simulink model "VFlexP"  (R2024a)
settings: Solver=ode23tb  StartTime=0.0  StopTime=3  FixedStep=1e-5
model workspace (MAT data in the model file):
  DCop_DCBUCK : object (value not decoded)
  Grid_CCVSC_idx = [2; 3; 4; 5; 6; 7; 8; 9; 10; 11; 12]
  Grid_CCVSCs = 1
  Grid_CCVSCs_buses = 1
  Grid_CCVSCs_toM = [0 1 0 0 0 0 0 0 0 0 0 0 ... (781 elements, 71x11)]
  Grid_C_Lines = [0 0]
  Grid_Cbuses = [0.00666666666667 0.00666666666667 0.00666666666667]
  Grid_DC : object (value not decoded)
  Grid_DCop_DCBUCK : object (value not decoded)
  Grid_DCop_DC_PES : object (value not decoded)
  Grid_DFIGs = 1
  Grid_DFIGs_buses = 1
  Grid_DGs : string (value not decoded)
  Grid_From_buses = [1 2]
  Grid_GFls = 1
  Grid_GFls_buses = 1
  Grid_GFr_idx = 1
  Grid_GFrs = 1
  Grid_GFrs_buses = 1
  Grid_GFrs_toM = [1; 0; 0]
  Grid_IG_idx = 2
  Grid_IGs = 1
  Grid_IGs_buses = 1
  Grid_IGs_toM = [0; 1]
  Grid_L_Lines = [0.05 0.05]
  Grid_L_Loads = 0
  Grid_Lines_fromM : object (value not decoded)
  Grid_Lines_toM : object (value not decoded)
  Grid_Load_buses = []
  Grid_Load_busesDC = []
  Grid_MSGs = 1
  Grid_MSGs_buses = 1
  Grid_Nbuses = 3
  Grid_PQ_gen = 3
  Grid_Ploads = []
  Grid_PloadsDC = []
  Grid_Ps_lf = -0.138475313333
  Grid_Qloads = []
  Grid_Qs_lf = 0.00594619333333
  Grid_R_Lines = [0.005 0.005]
  Grid_R_Loads = 0
  Grid_R_Loads_DC = 0
  Grid_Rcf = [150 150 150]
  Grid_SCs = 1
  Grid_SCs_buses = 1
  Grid_SG_idx = 1
  Grid_SGs = 1
  Grid_SGs_buses = 1
  Grid_SGs_toM = [1; 0]
  Grid_To_buses = [2 3]
  Grid_VCVSC_idx = [1; 2; 3; 4; 5; 6; 7; 8; 9; 10; 11; 12]
  Grid_VCVSCs = 1
  Grid_VCVSCs_buses = [1; 2; 3; 6; 8; 9; 12; 58; 59; 60; 63; 65]
  Grid_VCVSCs_toM = [1 0 0 0 0 0 0 0 0 0 0 0 ... (852 elements, 71x12)]
  Grid_VSM_idx = 2
  Grid_VSMs = 1
  Grid_VSMs_buses = 1
  Grid_VSMs_toM = [0; 1]
  Grid_admitt_matrix = [1.9801990198-19.801979198i  -1.9801980198+19.801980198i; -1.9801980198+19.801980198i  1.9801990198-19.801979198i]
  Grid_admitt_matrix_noloads = [1.9801990198-19.801979198i  -1.9801980198+19.801980198i; -1.9801980198+19.801980198i  1.9801990198-19.801979198i]
  Grid_bus = [1; 2; 3]
  Grid_busDC_complexity = 1
  Grid_busDC_complexity_PF = 2
  Grid_bus_complexity = [1 1 1]
  Grid_bus_complexity_PF = [1 1 1]
  Grid_buses_lf = 1
  Grid_conductance_matrix = 0.00666666666667
  Grid_conductance_matrix_noloads = 0.00666666666667
  Grid_fref : object (value not decoded)
  Grid_gen_static_params : mBase (value not decoded)
  Grid_iPs_lf = -7.22150378958
  Grid_iQs_lf = 168.17482109
  Grid_iadmitt_matrix = [250000.001075-249999.987531i  249999.998575-250000.012531i; 249999.998575-250000.012531i  250000.001075-249999.987531i]
  Grid_iadmitt_matrix_noloads = [250000.001075-249999.987531i  249999.998575-250000.012531i; 249999.998575-250000.012531i  250000.001075-249999.987531i]
  Grid_iconductance_matrix = 150
  Grid_iconductance_matrix_noloads = 150
  Grid_init_OK_bool = 1
  Grid_intconv_PF : object (value not decoded)
  Grid_lf_op : op_report (value not decoded)
  Grid_lineDC_complexity = []
  Grid_lineDC_complexity_PF = []
  Grid_line_complexity = [1 1]
  Grid_line_complexity_PF = [3 3]
  Grid_loadDC_complexity = []
  Grid_loadDC_complexity_PF = []
  Grid_load_complexity = []
  Grid_load_complexity_PF = []
  Grid_opDC_CCVSC : object (value not decoded)
  Grid_opDC_VSM : object (value not decoded)
  Grid_opGFr : object (value not decoded)
  Grid_opVCVSC : object (value not decoded)
  Grid_op_CCVSC : object (value not decoded)
  Grid_op_IG : object (value not decoded)
  Grid_op_SG : object (value not decoded)
  Grid_op_VSM : object (value not decoded)
  Grid_shift_lines = [0 0]
  Grid_tap_lines = [1 1]
  Grid_v_buses_mod = [1 1.0001218564 1]
  LinsysParamChangeStruct : Param1 (value not decoded)
  Lline = 0.01
  Rline = 1e-05
  linsys : object (value not decoded)
symbols that are objects in the model workspace (value not decoded): Grid_DCop_DC_PES, Grid_DCop_DCBUCK, Grid_op_CCVSC, Grid_op_IG, Grid_op_SG, Grid_op_VSM, Grid_opDC_CCVSC, Grid_opDC_VSM, Grid_opGFr, Grid_opVCVSC
undefined symbols (not defined in the file or in its folder): block_buses_DC, block_idx, CCVSC_idx, Cf, costs, costs2, DFIGs_nodes, DiscIntNeverNeededParam, entity, Fb, Fi, From_nodes, Grid_op_DFIG, Grid_op_DFIG_PQ, Grid_op_MSG, Grid_op_SC, Grid_op_VCVSC, Kic, Kiv, Kpc, Kpv, last_send, Lc, Lf, m, Matrix_flux_to_i, mD, mp, MSGs_buses, Nbuses_DC, nq, op_VCVSC, Psche, Rc, Rf, rkq1, rkq2, SCs_buses, SCs_nodes, sec_control_structure, set_DG_up, set_extra_satur, set_sending_cost, SGs_buses, SGs_nodes, Tf, To_nodes, VI_L, VI_R, WOF_Tf, xkq1, xkq2
libraries: simulink x447, eeGeneralControl x5
(part 5 of 30)

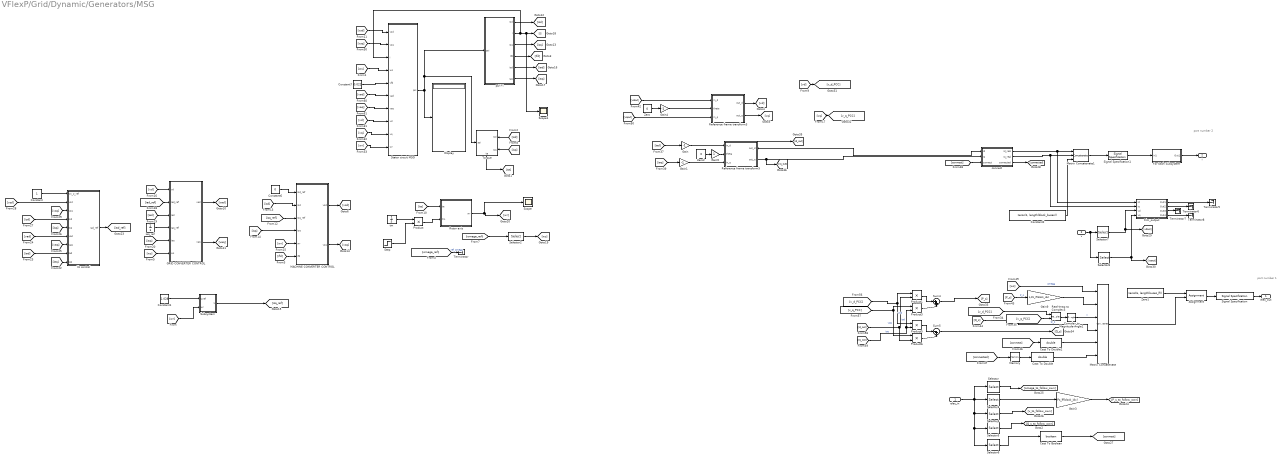
== system VFlexP/Grid/Dynamic/Generators/MSG ==
  note: port number 1
  note: port number 2
  elec_in : Inport
  v : Inport  Port=2
  Assignment : Assignment  NumberOfDimensions=2  DiagnosticForDimensions=Warning  IndexOptions=Assign all,Index vector (dialog)  Indices=1,block_idx  OutputSizes=1,1
  Cast To Boolean : DataTypeConversion  OutDataTypeStr=boolean  SaturateOnIntegerOverflow=off  RndMeth=Floor
  Cast To Double : DataTypeConversion  OutDataTypeStr=double  SaturateOnIntegerOverflow=off  RndMeth=Floor
  Cast To Double1 : DataTypeConversion  OutDataTypeStr=double  SaturateOnIntegerOverflow=off  RndMeth=Floor
  Complex to Magnitude-Angle1 : ComplexToMagnitudeAngle  Output=Magnitude
  Constant : Constant
  Constant1 : Constant  Value=1.028
  Constant2 : Constant  Value=zeros(1, length(block_buses))  VectorParams1D=off
  Constant6 : Constant  Value=0
  Constant7 : Constant  Value=0.022
  Display : Display
  For Each Subsystem : Subsystem  TreatAsAtomicUnit=on
  GRID CONVERTER CONTROL : Subsystem
  Gain : Gain  Gain=-1
  Gain1 : Gain  Gain=-1
  Gain3 : Gain  Gain=Ps_lf(block_idx)
  Gain4 : Gain  Gain=-1
  Gain5 : Gain
  Gain9 : Gain  Gain=1./Ps_lf(block_idx)
  MACHINE CONVERTER CONTROL : Subsystem
  Matrix Concatenate : Concatenate  NumInputs=6  Mode=Multidimensional array
  Matrix Concatenate1 : Concatenate  NumInputs=3  Mode=Multidimensional array
  Memory : Memory  InitialCondition=1
  Product{,1,3,5..6} (5 alike) : Product
  Real-Imag to Complex3 : RealImagToComplex
  Reference frame transform3 : Subsystem
  Reference frame transform5 : Subsystem
  Rotor axis : Subsystem
  Scope : Scope
  Scope1 : Scope
  Selector : Selector  NumberOfDimensions=2  InputPortWidth=3  IndexOptions=Index vector (dialog),Index vector (dialog)  Indices=1,block_idx  OutputSizes=1,1
  Selector2 : Selector  InputPortWidth=length(fref.ref_units)  IndexOptions=Index vector (dialog)  Indices=block_fref  OutputSizes=1
  Selector3 : Selector  NumberOfDimensions=2  InputPortWidth=3  IndexOptions=Index vector (dialog),Index vector (dialog)  Indices=2,block_idx  OutputSizes=1,1
  Selector4 : Selector  NumberOfDimensions=2  InputPortWidth=3  IndexOptions=Index vector (dialog),Index vector (dialog)  Indices=3,block_idx  OutputSizes=1,1
  Selector5 : Selector  NumberOfDimensions=2  InputPortWidth=3  IndexOptions=Index vector (dialog),Index vector (dialog)  Indices=4,block_idx  OutputSizes=1,1
  Selector6 : Selector  NumberOfDimensions=2  InputPortWidth=3  IndexOptions=Index vector (dialog),Index vector (dialog)  Indices=5,block_idx  OutputSizes=1,1
  Selector7 : Selector  NumberOfDimensions=2  InputPortWidth=3  IndexOptions=Index vector (dialog),Index vector (dialog)  Indices=1,block_buses  OutputSizes=1,1
  Selector8 : Selector  NumberOfDimensions=2  InputPortWidth=3  IndexOptions=Index vector (dialog),Index vector (dialog)  Indices=2,block_buses  OutputSizes=1,1
  Signal Specification : SignalSpecification  Dimensions=[6 length(buses_lf)]
  Signal Specification1 : SignalSpecification  Dimensions=[3 length(block_buses)]
  Stator circuit MSG : Subsystem
  Step : Step  Before=1  After=1.1  SampleTime=0
  Subsystem : Subsystem
  Sum4 : Sum  Inputs=|++
  Sum5 : Sum  Inputs=|-+
  Terminator{,5..8} (5 alike) : Terminator
  Torque : Subsystem
      settings: PortSchema="{\"entries\":[{\"content\":{\"sides\":[{\"content\":{\"connectorIds\":[\"In1\"]},\"type\":\"ConnectorPlacement.EquallySpacedRectSide\",\"uuid\":\"b7abd3bc-22dd-4669-aa40-98bc76884565\"},{\"content\":{\"connectorIds\":[\"In2\",\"In3\"],\"side\":\"RIGHT\"},\"type\":\"ConnectorPlacement.EquallySpacedRectSide\",\"uuid\":\"e9abb552-b46d-48ed-aa1f-0e9dac604fea\"},{\"content\":{\"connectorIds\":[],\"side\":\"TOP\"},\"type\":\"ConnectorPlacement.EquallySpacedRectSide\",\"uuid\":\"4b14997d-8f32-4cfb-8a1b-18cffb093d28\"},{\"content\":{\"connectorIds\":[\"Out1\"],\"side\":\"BOTTOM\"},\"type\":\"ConnectorPlacement.EquallySpacedRectSide\",\"uuid\":\"0ad577f8-eb9c-4d21-85f4-8d3c6640245c\"}]},\"type\":\"ConnectorPlacement.EquallySpacedConnector\",\"uuid\":\"d6624493-e930-4f0d-8cbe-17f96cb72edc\"}],\"packageUris\":[\"http://schema.mathworks.com/mf0/Connector/R2020b\"],\"version\":\"1.0\"}"
  Vc control : Subsystem
  Zero : Constant  Value=0  OutDataTypeStr=Inherit: Inherit via back propagation
  Zero1 : Constant  Value=zeros(6, length(buses_lf))  VectorParams1D=off  OutDataTypeStr=Inherit: Inherit via back propagation
  Zero2 : Constant  Value=0  OutDataTypeStr=Inherit: Inherit via back propagation
  connect : Subsystem
  iaq_ref : Integrator  InitialCondition=Grid_op_MSG.op.States(14).x'
  psi->i : Subsystem
  tm : Integrator  InitialCondition=Grid_op_MSG.op.States(15).x'
  trim_output : Subsystem
  elec_out : Outport
  i : Outport  Port=2
  wires:
  Product5/1 -> Sum5/1
  [v_d_PCC] -> Product1/1, Product5/1  "vod"
  Product3/1 -> Sum4/2
  [id_out] -> Product1/2, Product6/2  "iod"
  Sum5/1 -> [Q_s]
  [v_q_PCC] -> Product6/1, Product3/1  "voq"
  Product6/1 -> Sum5/2
  Sum4/1 -> [P_s]
  Product1/1 -> Sum4/1
  [iq_out] -> Product3/2, Product5/2  "ioq"
  Signal Specification/1 -> elec_out/1
  Gain4/1 -> Reference frame transform3/2(theta)
  For Each Subsystem/1(Out1) -> i/1
  [omega_ref] -> Selector2/1
  trim_output/2(Out2) -> Terminator6/1
  Selector5/1 -> [Q_s_to_follow_own]
  [iad] -> GRID CONVERTER CONTROL/3(iad)
  Vc control/1(iad_ref) -> [iad_ref]
  [vsd] -> Vc control/2(vsd)
  [vad] -> Vc control/6(vad)
  [te] -> Rotor axis/1(te)
  [omega_ref] -> Terminator/1  "ref_omega"
  Assignment/1 -> Signal Specification/1
  GRID CONVERTER CONTROL/1(vad) -> [vad]
  [iaq] -> Vc control/9(iaq)
  GRID CONVERTER CONTROL/2(vaq) -> [vaq]
  [vsq] -> Vc control/3(vsq)
  psi->i/3(isq) -> [isq]
  [iad_ref] -> GRID CONVERTER CONTROL/2(iad_ref)
  Constant/1 -> Vc control/1(Vc_2_ref)
  iaq_ref/1 -> GRID CONVERTER CONTROL/4(iaq_ref)
  [iad] -> Vc control/8(iad)
  [vdout] -> Reference frame transform3/1(in_d)
  Zero/1 -> Gain4/1
  Gain9/1 -> Matrix Concatenate/2
  [P_s] -> Gain9/1  "P_s"
  Matrix Concatenate1/1 -> Signal Specification1/1
  trim_output/4(Out4) -> Terminator8/1
  Selector8/1 -> [vqout], trim_output/4(vq)
  Constant2/1 -> Matrix Concatenate1/3
  trim_output/3(Out3) -> Terminator7/1
  Cast To Boolean/1 -> [connect]
  v/1 -> Selector8/1, Selector7/1
  Signal Specification1/1 -> For Each Subsystem/1(In1)
  [vd] -> GRID CONVERTER CONTROL/1(vd)
  [ws] -> GRID CONVERTER CONTROL/6(ws)
  Selector7/1 -> trim_output/3(vd), [vdout]
  Gain5/1 -> Reference frame transform5/2(theta)
  elec_in/1 -> Selector6/1, Selector5/1, Selector4/1, Selector3/1, Selector/1
  connect/2(iq_real) -> trim_output/2(iq), Matrix Concatenate1/2
  [connect] -> Cast To Double1/1
  Cast To Double/1 -> Matrix Concatenate/6
  Cast To Double1/1 -> Matrix Concatenate/5
  Selector6/1 -> Cast To Boolean/1
  [Q_s] -> Matrix Concatenate/4  "Q_s"
  connect/1(id_real) -> trim_output/1(id), Matrix Concatenate1/1
  psi->i/2(i) -> Stator circuit MSG/3(i), Scope1/1, [i]
  trim_output/1(Out1) -> Terminator5/1
  [ws] -> Matrix Concatenate/1  "omega"
  Zero1/1 -> Assignment/1
  Selector/1 -> [omega_to_follow_own]
  Selector3/1 -> Gain3/1
  Selector4/1 -> [v_to_follow_own]
  Gain3/1 -> [P_s_to_follow_own]
  [vaq] -> Vc control/7(vaq)
  [isd] -> Vc control/4(isd)
  Matrix Concatenate/1 -> Assignment/2
  [iaq] -> GRID CONVERTER CONTROL/5(iaq)
  Zero2/1 -> Gain5/1
  psi->i/1(isd) -> [isd]
  [connect] -> connect/3(connect)
  [iad] -> Gain/1
  [connected] -> Memory/1
  [isq] -> Vc control/5(isq)
  connect/3(connected) -> [connected]
  Memory/1 -> Cast To Double/1
  Stator circuit MSG/1(psi) -> Torque/1(psi), psi->i/1(psi), Display/1
  Rotor axis/1(wr) -> Scope/1, [wr]
  Constant6/1 -> MACHINE CONVERTER CONTROL/1(isd_ref)
  [isq_ref] -> MACHINE CONVERTER CONTROL/3(isq_ref)
  MACHINE CONVERTER CONTROL/1(vsd) -> [vsd]
  [wr] -> MACHINE CONVERTER CONTROL/5(wr)
  MACHINE CONVERTER CONTROL/2(vsq) -> [vsq]
  Constant1/1 -> Subsystem/1(wref)
  [wr] -> Subsystem/2(wr)
  [ifd] -> MACHINE CONVERTER CONTROL/6(ifd)
  [vsd] -> Stator circuit MSG/1(vsd)
  [vsq] -> Stator circuit MSG/2(vsq)
  [vad] -> Stator circuit MSG/6(vad)
  [vaq] -> Stator circuit MSG/7(vaq)
  [ws] -> Stator circuit MSG/4(ws)
  [isd] -> Torque/2(isd)
  [isq] -> Torque/3(isq)
  Torque/1(te) -> [te]
  [vd] -> Stator circuit MSG/8(vd)
  [vq] -> Stator circuit MSG/9(vq)
  [wr] -> Stator circuit MSG/10(wr)
  [iaq] -> Gain1/1
  [v_q_PCC] -> Real-Imag to Complex3/2
  Real-Imag to Complex3/1 -> Complex to Magnitude-Angle1/1
  Complex to Magnitude-Angle1/1 -> Matrix Concatenate/3  "v"
  [v_d_PCC] -> Real-Imag to Complex3/1
  psi->i/5(iad) -> [iad]
  psi->i/6(iaq) -> [iaq]
  [vqout] -> Reference frame transform3/3(in_q)
  psi->i/4(ifd) -> [ifd]
  Constant7/1 -> Stator circuit MSG/5(vfd)
  Reference frame transform3/1(out_d) -> [vd]
  [vd] -> [v_d_PCC]
  Reference frame transform3/2(out_q) -> [vq]
  [vq] -> [v_q_PCC]
  Gain/1 -> Reference frame transform5/1(in_d)
  Gain1/1 -> Reference frame transform5/3(in_q)
  Reference frame transform5/1(out_d) -> [id_out], connect/1(id)
  Reference frame transform5/2(out_q) -> [iq_out], connect/2(iq)
  Subsystem/1(isq_ref) -> [isq_ref]
  [isd] -> MACHINE CONVERTER CONTROL/2(isd)
  [isq] -> MACHINE CONVERTER CONTROL/4(isq)
  tm/1 -> Product/1
  Step/1 -> Product/2
  Product/1 -> Rotor axis/2(tm)
  Selector2/1 -> [ws]

== system VFlexP/Grid/Dynamic/Generators/SC ==
  note: AVR
  note: do not rename this block, conditions to initialise the generator from PF result are set on this block's output
  note: port number 1
  note: port number 2
  elec_in : Inport
  v : Inport  Port=2
  AVR_Exciter : Subsystem  mask{T_s=T_e}
      mask prompts: T_s "Filter time constant"
      mask Display:
      | try
      |     dpoly(1, [T_s, 1])
      | catch
      | end
  AVR_LeadLag : Subsystem  mask{T_2=T_2, T_1=T_1}
      mask help:
      | Transfer function:
      |
      |   1 + sT_2
      | ---------------
      |   1 + sT_1
      mask Display:
      | try
      |     dpoly([T_2, 1], [T_1, 1])
      | catch
      | end
  AVR_MainRegulator : Subsystem  mask{T_s=T_A}
      mask prompts: T_s "Filter time constant"
      mask Display:
      | try
      |     dpoly(1, [T_s, 1])
      | catch
      | end
  AVR_Vmeas_Filter : Subsystem  mask{T_r=0.01}
      mask prompts: T_r "Filter time constant"
      mask Display:
      | try
      |     dpoly(1, [T_r, 1])
      | catch
      | end
  Abs : Abs  SaturateOnIntegerOverflow=off
  Assignment : Assignment  NumberOfDimensions=2  DiagnosticForDimensions=Warning  IndexOptions=Assign all,Index vector (dialog)  Indices=1,block_idx  OutputSizes=1,1
  Cast To Boolean : DataTypeConversion  OutDataTypeStr=boolean  SaturateOnIntegerOverflow=off  RndMeth=Floor
  Cast To Double : DataTypeConversion  OutDataTypeStr=double  SaturateOnIntegerOverflow=off  RndMeth=Floor
  Cast To Double1 : DataTypeConversion  OutDataTypeStr=double  SaturateOnIntegerOverflow=off  RndMeth=Floor
  Constant : Constant  Value=zeros(1, length(block_buses))  VectorParams1D=off
  For Each Subsystem : Subsystem  TreatAsAtomicUnit=on
  Gain1 : Gain  Gain=0.01
  Gain2 : Gain  Gain=-1
  Gain4 : Gain  Gain=3.4e-4
  Gain7 : Gain  Gain=0.001
  Gain8 : Gain  Gain=K_A
  Gain9 : Gain
  Integrator1 : Integrator  InitialCondition=Grid_op_SC.op.States(5).x'
  Integrator2 : Integrator  InitialCondition=Grid_op_SC.op.States(6).x'
  Integrator3 : Integrator  InitialCondition=Grid_op_SC.op.States(7).x'
  Matrix Concatenate : Concatenate  NumInputs=6  Mode=Multidimensional array
  Matrix Concatenate1 : Concatenate  NumInputs=3  Mode=Multidimensional array
  Memory : Memory  InitialCondition=1
  Memory1 : Memory  InitialCondition=1
  Memory2 : Memory  InitialCondition=1
  Product{,1..4} (5 alike) : Product
  Real-Imag to Complex : RealImagToComplex
  Reference frame transform1 : Subsystem
  Reference frame transform2 : Subsystem
  Rotor axis : Subsystem
  Selector : Selector  NumberOfDimensions=2  InputPortWidth=3  IndexOptions=Index vector (dialog),Index vector (dialog)  Indices=1,block_idx  OutputSizes=1,1
  Selector1 : Selector  NumberOfDimensions=2  InputPortWidth=3  IndexOptions=Index vector (dialog),Index vector (dialog)  Indices=2,block_idx  OutputSizes=1,1
  Selector2 : Selector  NumberOfDimensions=2  InputPortWidth=3  IndexOptions=Index vector (dialog),Index vector (dialog)  Indices=3,block_idx  OutputSizes=1,1
  Selector3 : Selector  NumberOfDimensions=2  InputPortWidth=3  IndexOptions=Index vector (dialog),Index vector (dialog)  Indices=4,block_idx  OutputSizes=1,1
  Selector4 : Selector  NumberOfDimensions=2  InputPortWidth=3  IndexOptions=Index vector (dialog),Index vector (dialog)  Indices=5,block_idx  OutputSizes=1,1
  Selector5 : Selector  NumberOfDimensions=2  InputPortWidth=3  IndexOptions=Index vector (dialog),Index vector (dialog)  Indices=1,block_buses  OutputSizes=1,1
  Selector6 : Selector  NumberOfDimensions=2  InputPortWidth=3  IndexOptions=Index vector (dialog),Index vector (dialog)  Indices=2,block_buses  OutputSizes=1,1
  Selector7 : Selector  InputPortWidth=length(fref.ref_units)  IndexOptions=Index vector (dialog)  Indices=block_fref  OutputSizes=1
  Selector8 : Selector  InputPortWidth=length(fref.ref_units)  IndexOptions=Index vector (dialog)  Indices=block_fref  OutputSizes=1
  Signal Specification : SignalSpecification  Dimensions=[6 length(buses_lf)]
  Signal Specification1 : SignalSpecification  Dimensions=[3 length(block_buses)]
  Stator circuit : Subsystem
  Sum1 : Sum  Inputs=|-+
  Sum2 : Sum  Inputs=|+-
  Sum4 : Sum  Inputs=|-+
  Sum5 : Sum  Inputs=|++
  Sum8 : Sum  Inputs=|-+
  Sum9 : Sum  Inputs=|++
  Terminator{2..5} (4 alike) : Terminator
  Torque : Subsystem
      settings: PortSchema="{\"entries\":[{\"content\":{\"sides\":[{\"content\":{\"connectorIds\":[\"In1\"]},\"type\":\"ConnectorPlacement.EquallySpacedRectSide\",\"uuid\":\"b7abd3bc-22dd-4669-aa40-98bc76884565\"},{\"content\":{\"connectorIds\":[\"In2\",\"In3\",\"Out1\"],\"side\":\"RIGHT\"},\"type\":\"ConnectorPlacement.EquallySpacedRectSide\",\"uuid\":\"e9abb552-b46d-48ed-aa1f-0e9dac604fea\"},{\"content\":{\"connectorIds\":[],\"side\":\"TOP\"},\"type\":\"ConnectorPlacement.EquallySpacedRectSide\",\"uuid\":\"4b14997d-8f32-4cfb-8a1b-18cffb093d28\"}]},\"type\":\"ConnectorPlacement.EquallySpacedConnector\",\"uuid\":\"d6624493-e930-4f0d-8cbe-17f96cb72edc\"}],\"packageUris\":[\"http://schema.mathworks.com/mf0/Connector/R2020b\"],\"version\":\"1.0\"}"
  Transport Delay : TransportDelay  DelayTime=0.0001  TransDelayFeedthrough=on
  Zero1 : Constant  Value=zeros(6, length(buses_lf))  VectorParams1D=off  OutDataTypeStr=Inherit: Inherit via back propagation
  connect : Subsystem
  psi->i : Subsystem
  theta : Integrator  InitialCondition=Grid_op_SC.op.States(17).x'  UpperSaturationLimit=2*pi  LowerSaturationLimit=0
  trim_output : Subsystem
  elec_out : Outport
  i : Outport  Port=2
  wires:
  Sum4/1 -> [Qe]
  Sum5/1 -> [Pe]
  [v_q_PCC] -> Real-Imag to Complex/2
  Real-Imag to Complex/1 -> Abs/1
  [v_d_PCC] -> Real-Imag to Complex/1
  [vqout] -> Product3/1, Product1/2
  [iq] -> Product3/2, Product/2
  Product/1 -> Sum4/1
  Product1/1 -> Sum4/2
  theta/1 -> [theta]
  psi->i/1(isd) -> Reference frame transform1/1(in_d), Torque/2(isd), [isd]
  psi->i/3(isq) -> [isq], Torque/3(isq), Reference frame transform1/3(in_q)
  Stator circuit/1(psi) -> Torque/1(psi), psi->i/1(psi)
  [v_q_PCC] -> Stator circuit/2(vsq)
  Gain2/1 -> Reference frame transform1/2(theta)
  Rotor axis/1(wr) -> Stator circuit/4(ws), Sum1/1, [omega]
  Torque/1(te) -> Rotor axis/1(te)
  [theta] -> Gain2/1
  psi->i/2(i) -> Stator circuit/3(i)
  [vdout] -> Product/1, Product2/1
  Product3/1 -> Sum5/2
  [omega_ref] -> Selector7/1  "ref_omega"
  Product2/1 -> Sum5/1
  [id] -> Product2/2, Product1/1
  [v_d_PCC] -> Stator circuit/1(vsd)
  Integrator2/1 -> Rotor axis/2(tm)
  Gain9/1 -> AVR_Exciter/1(in)
  AVR_Exciter/1(out) -> Gain4/1
  Sum2/1 -> Gain8/1
  AVR_LeadLag/1(Out1) -> Gain9/1
  Gain8/1 -> AVR_MainRegulator/1(in)
  AVR_MainRegulator/1(out) -> AVR_LeadLag/1(In1)
  Selector3/1 -> [Q_s_to_follow_own]
  Selector/1 -> [omega_to_follow_own]
  Selector2/1 -> [v_to_follow_own]
  Selector1/1 -> Transport Delay/1
  [Qe] -> Matrix Concatenate/4  "Q_s"
  [Pe] -> Matrix Concatenate/2  "P_s"
  Abs/1 -> Matrix Concatenate/3, AVR_Vmeas_Filter/1(in)  "v"
  [omega] -> Matrix Concatenate/1  "omega"
  Cast To Double/1 -> Matrix Concatenate/6
  [connected] -> Memory/1
  Cast To Double1/1 -> Matrix Concatenate/5
  [connect] -> Memory1/1
  [connect] -> connect/3(connect)
  connect/3(connected) -> [connected]
  connect/2(iq_real) -> Matrix Concatenate1/2, trim_output/2(iq), [iq]
  connect/1(id_real) -> Matrix Concatenate1/1, trim_output/1(id), [id]
  Cast To Boolean/1 -> [connect]
  Selector4/1 -> Memory2/1
  Sum8/1 -> Gain1/1, Gain7/1
  [Qe] -> Sum8/1
  Integrator3/1 -> Sum9/2
  Gain7/1 -> Sum9/1
  [Q_s_to_follow_own] -> Sum8/2
  Zero1/1 -> Assignment/1
  Signal Specification/1 -> elec_out/1
  elec_in/1 -> Selector4/1, Selector3/1, Selector2/1, Selector1/1, Selector/1
  Assignment/1 -> Signal Specification/1
  Matrix Concatenate/1 -> Assignment/2
  Matrix Concatenate1/1 -> Signal Specification1/1
  Signal Specification1/1 -> For Each Subsystem/1(In1)
  Constant/1 -> Matrix Concatenate1/3
  For Each Subsystem/1(Out1) -> i/1
  trim_output/1(Out1) -> Terminator2/1
  trim_output/2(Out2) -> Terminator3/1
  trim_output/4(Out4) -> Terminator5/1
  Selector5/1 -> trim_output/3(vd), [vdout]
  Selector6/1 -> [vqout], trim_output/4(vq)
  trim_output/3(Out3) -> Terminator4/1
  v/1 -> Selector6/1, Selector5/1
  Reference frame transform1/1(out_d) -> connect/1(id)
  Reference frame transform1/2(out_q) -> connect/2(iq)
  Gain1/1 -> Integrator3/1
  Memory/1 -> Cast To Double/1
  Memory1/1 -> Cast To Double1/1
  Memory2/1 -> Cast To Boolean/1
  Transport Delay/1 -> [P_s_to_follow_own]
  Reference frame transform2/1(out_d) -> [v_d_PCC]
  Reference frame transform2/2(out_q) -> [v_q_PCC]
  [theta] -> Reference frame transform2/2(theta)
  [vqout] -> Reference frame transform2/3(in_q)
  [vdout] -> Reference frame transform2/1(in_d)
  AVR_Vmeas_Filter/1(out) -> Sum2/2
  Gain4/1 -> Stator circuit/5(vfd)
  Integrator1/1 -> Sum2/1
  [omega_base] -> Selector8/1
  Selector8/1 -> Product4/2
  Product4/1 -> theta/1
  Sum1/1 -> Product4/1
  Selector7/1 -> Sum1/2

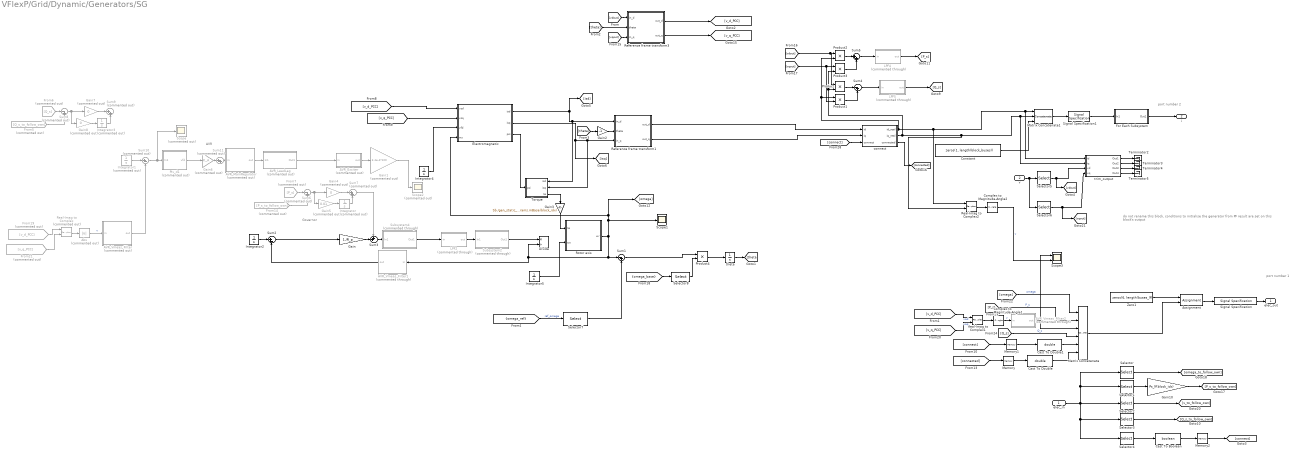
== system VFlexP/Grid/Dynamic/Generators/SG ==
  note: Governor
  note: do not rename this block, conditions to initialise the generator from PF result are set on this block's output
  note: port number 1
  note: port number 2
  note: AVR
  elec_in : Inport
  v : Inport  Port=2
  AVR_Exciter : Subsystem  Commented=on  mask{T_s=T_e}
      mask prompts: T_s "Filter time constant"
      mask Display:
      | try
      |     dpoly(1, [T_s, 1])
      | catch
      | end
  AVR_LeadLag : Subsystem  Commented=on  mask{T_2=T_2, T_1=T_1}
      mask help:
      | Transfer function:
      |
      |   1 + sT_2
      | ---------------
      |   1 + sT_1
      mask Display:
      | try
      |     dpoly([T_2, 1], [T_1, 1])
      | catch
      | end
  AVR_MainRegulator : Subsystem  Commented=on  mask{T_s=T_A}
      mask prompts: T_s "Filter time constant"
      mask Display:
      | try
      |     dpoly(1, [T_s, 1])
      | catch
      | end
  AVR_Vmeas_Filter : Subsystem  Commented=on  mask{T_r=0.01}
      mask prompts: T_r "Filter time constant"
      mask Display:
      | try
      |     dpoly(1, [T_r, 1])
      | catch
      | end
  AVR_Vmeas_Filter1 : Subsystem  Commented=through  mask{T_r=0.01}
      mask prompts: T_r "Filter time constant"
      mask Display:
      | try
      |     dpoly(1, [T_r, 1])
      | catch
      | end
  AVR_Vmeas_Filter2 : Subsystem  Commented=through  mask{T_r=0.01}
      mask prompts: T_r "Filter time constant"
      mask Display:
      | try
      |     dpoly(1, [T_r, 1])
      | catch
      | end
  Abs : Abs  Commented=on  SaturateOnIntegerOverflow=off
  Assignment : Assignment  NumberOfDimensions=2  DiagnosticForDimensions=Warning  IndexOptions=Assign all,Index vector (dialog)  Indices=1,block_idx  OutputSizes=1,1
  Cast To Boolean : DataTypeConversion  OutDataTypeStr=boolean  SaturateOnIntegerOverflow=off  RndMeth=Floor
  Cast To Double : DataTypeConversion  OutDataTypeStr=double  SaturateOnIntegerOverflow=off  RndMeth=Floor
  Cast To Double1 : DataTypeConversion  OutDataTypeStr=double  SaturateOnIntegerOverflow=off  RndMeth=Floor
  Complex to Magnitude-Angle1 : ComplexToMagnitudeAngle  Output=Magnitude
  Complex to Magnitude-Angle2 : ComplexToMagnitudeAngle  Output=Magnitude
  Constant : Constant  Value=zeros(1, length(block_buses))  VectorParams1D=off
  Divide : Product  Inputs=*/
  Electromagnetic : Subsystem  Variant=on  VariantControlMode=label  LabelModeActiveChoice=order 2
  For Each Subsystem : Subsystem  TreatAsAtomicUnit=on
  From14 : From  Commented=on  GotoTag=P_s_to_follow_own
  From19 : From  Commented=on  GotoTag=v_d_PCC
  From21 : From  Commented=on  GotoTag=v_q_PCC
  From5 : From  Commented=on  GotoTag=Q_s_to_follow_own
  From6 : From  Commented=on  GotoTag=Q_s
  From7 : From  Commented=on  GotoTag=P_s
  Gain : Gain  Gain=1./R_p
  Gain1 : Gain  Commented=on  Gain=3.4e-4*100
  Gain10 : Gain  Gain=Ps_lf(block_idx)
  Gain2 : Gain  Gain=-1
  Gain3 : Gain  Gain=Sb./gen_static_params.mBase(block_idx)
  Gain4 : Gain  Commented=on  Gain=0
  Gain5 : Gain  Commented=on  Gain=0.01
  Gain6 : Gain  Commented=on  Gain=K_A
  Gain7 : Gain  Commented=on  Gain=0
  Gain8 : Gain  Commented=on  Gain=0
  Integrator : Integrator  Commented=on  InitialCondition=Grid_op_SG.op.States(1).x'
  Integrator1 : Integrator  Commented=on  InitialCondition=Grid_op_SG.op.States(8).x'
  Integrator2 : Integrator  InitialCondition=Grid_op_SG.op.States(4).x'
  Integrator3 : Integrator  Commented=on  InitialCondition=Grid_op_SG.op.States(2).x'
  Integrator4 : Integrator  InitialCondition=Grid_op_SG.op.States(5).x'
  Integrator5 : Integrator  InitialCondition=Grid_op_SG.op.States(6).x'
  LPF2 : Subsystem  Commented=through  mask{T_s=T_g}
      mask prompts: T_s "Filter time constant"
      mask Display:
      | try
      |     dpoly(1, [T_s, 1])
      | catch
      | end
  LPF4 : Subsystem  Commented=through  mask{T_s=0.01}
      mask prompts: T_s "Filter time constant"
      mask Display:
      | try
      |     dpoly(1, [T_s, 1])
      | catch
      | end
  LPF5 : Subsystem  Commented=through  mask{T_s=0.01}
      mask prompts: T_s "Filter time constant"
      mask Display:
      | try
      |     dpoly(1, [T_s, 1])
      | catch
      | end
  Matrix Concatenate : Concatenate  NumInputs=6  Mode=Multidimensional array
  Matrix Concatenate1 : Concatenate  NumInputs=3  Mode=Multidimensional array
  Memory : Memory  InitialCondition=1
  Memory1 : Memory  InitialCondition=1
  Memory2 : Memory  InitialCondition=1
  PIv_d1 : Subsystem  Commented=on
  Product{,1..4} (5 alike) : Product
  Real-Imag to Complex : RealImagToComplex  Commented=on
  Real-Imag to Complex1 : RealImagToComplex
  Real-Imag to Complex2 : RealImagToComplex
  Reference frame transform1 : Subsystem
  Reference frame transform3 : Subsystem
  Rotor axis : Subsystem
  Scope : Scope  Commented=on
  Scope1 : Scope
  Scope2 : Scope  Commented=on
  Scope3 : Scope  NumInputPorts=2
  Selector : Selector  NumberOfDimensions=2  InputPortWidth=3  IndexOptions=Index vector (dialog),Index vector (dialog)  Indices=1,block_idx  OutputSizes=1,1
  Selector1 : Selector  NumberOfDimensions=2  InputPortWidth=3  IndexOptions=Index vector (dialog),Index vector (dialog)  Indices=2,block_idx  OutputSizes=1,1
  Selector2 : Selector  NumberOfDimensions=2  InputPortWidth=3  IndexOptions=Index vector (dialog),Index vector (dialog)  Indices=3,block_idx  OutputSizes=1,1
  Selector3 : Selector  NumberOfDimensions=2  InputPortWidth=3  IndexOptions=Index vector (dialog),Index vector (dialog)  Indices=4,block_idx  OutputSizes=1,1
  Selector4 : Selector  NumberOfDimensions=2  InputPortWidth=3  IndexOptions=Index vector (dialog),Index vector (dialog)  Indices=5,block_idx  OutputSizes=1,1
  Selector5 : Selector  NumberOfDimensions=2  InputPortWidth=3  IndexOptions=Index vector (dialog),Index vector (dialog)  Indices=1,block_buses  OutputSizes=1,1
  Selector6 : Selector  NumberOfDimensions=2  InputPortWidth=3  IndexOptions=Index vector (dialog),Index vector (dialog)  Indices=2,block_buses  OutputSizes=1,1
  Selector7 : Selector  InputPortWidth=length(fref.ref_units)  IndexOptions=Index vector (dialog)  Indices=block_fref  OutputSizes=1
  Selector8 : Selector  InputPortWidth=length(fref.ref_units)  IndexOptions=Index vector (dialog)  Indices=block_fref  OutputSizes=1
  Signal Specification : SignalSpecification  Dimensions=[6 length(buses_lf)]
  Signal Specification1 : SignalSpecification  Dimensions=[3 length(block_buses)]
  Subsystem2 : Subsystem  Commented=through  mask{T_2=-T_W, T_1=0.5*T_W}
      mask help:
      | Transfer function:
      |
      |   1 + sT_2
      | ---------------
      |   1 + sT_1
      mask Display:
      | try
      |     dpoly([T_2, 1], [T_1, 1])
      | catch
      | end
  Subsystem4 : Subsystem  Commented=through  mask{T_2=T_R, T_1=T_R*(R_t/R_p)}
      mask help:
      | Transfer function:
      |
      |   1 + sT_2
      | ---------------
      |   1 + sT_1
      mask Display:
      | try
      |     dpoly([T_2, 1], [T_1, 1])
      | catch
      | end
  Sum1 : Sum  Inputs=|-+
  Sum10 : Sum  Commented=on  Inputs=|+-
  Sum11 : Sum  Commented=on  Inputs=|++
  Sum2 : Sum  Inputs=|+-
  Sum3 : Sum  Inputs=++|
  Sum4 : Sum  Inputs=|-+
  Sum5 : Sum  Inputs=|++
  Sum6 : Sum  Commented=on  Inputs=|-+
  Sum7 : Sum  Commented=on  Inputs=|++
  Sum8 : Sum  Commented=on  Inputs=|-+
  Sum9 : Sum  Commented=on  Inputs=|++
  Terminator{2..5} (4 alike) : Terminator
  Torque : Subsystem
      settings: PortSchema="{\"entries\":[{\"content\":{\"sides\":[{\"content\":{\"connectorIds\":[\"In1\"]},\"type\":\"ConnectorPlacement.EquallySpacedRectSide\",\"uuid\":\"b7abd3bc-22dd-4669-aa40-98bc76884565\"},{\"content\":{\"connectorIds\":[\"In2\",\"In3\",\"Out1\"],\"side\":\"RIGHT\"},\"type\":\"ConnectorPlacement.EquallySpacedRectSide\",\"uuid\":\"e9abb552-b46d-48ed-aa1f-0e9dac604fea\"},{\"content\":{\"connectorIds\":[],\"side\":\"TOP\"},\"type\":\"ConnectorPlacement.EquallySpacedRectSide\",\"uuid\":\"4b14997d-8f32-4cfb-8a1b-18cffb093d28\"}]},\"type\":\"ConnectorPlacement.EquallySpacedConnector\",\"uuid\":\"d6624493-e930-4f0d-8cbe-17f96cb72edc\"}],\"packageUris\":[\"http://schema.mathworks.com/mf0/Connector/R2020b\"],\"version\":\"1.0\"}"
  Zero1 : Constant  Value=zeros(6, length(buses_lf))  VectorParams1D=off  OutDataTypeStr=Inherit: Inherit via back propagation
  connect : Subsystem
  theta : Integrator  InitialCondition=Grid_op_SG.op.States(8).x'  UpperSaturationLimit=2*pi  LowerSaturationLimit=0
  trim_output : Subsystem
  elec_out : Outport
  i : Outport  Port=2
  wires:
  LPF5/1(out) -> [Q_s]
  Reference frame transform1/2(out_q) -> connect/2(iq)
  Product/1 -> Sum4/1
  Product1/1 -> Sum4/2
  theta/1 -> [theta]
  Gain2/1 -> Reference frame transform1/2(theta)
  [theta] -> Reference frame transform3/2(theta)
  Subsystem2/1(Out1) -> Divide/1
  [theta] -> Gain2/1
  LPF2/1(out) -> Subsystem2/1(In1)
  Sum4/1 -> LPF5/1(in)
  Sum5/1 -> LPF4/1(in)
  Product3/1 -> Sum5/2
  [omega_ref] -> Selector7/1  "ref_omega"
  From7/1 -> Sum6/1
  Gain/1 -> Sum3/2
  Product2/1 -> Sum5/1
  Reference frame transform1/1(out_d) -> connect/1(id)
  Sum6/1 -> Gain4/1, Gain5/1
  Integrator/1 -> Sum7/2
  Gain4/1 -> Sum7/1
  Gain5/1 -> Integrator/1
  Subsystem4/1(Out1) -> LPF2/1(in)
  LPF4/1(out) -> [P_s]
  Integrator2/1 -> Sum2/1
  Rotor axis/1(wr) -> Electromagnetic/4(ws), [omega], Scope1/1, Sum1/1, Divide/2, AVR_Vmeas_Filter1/1(in)
  [P_s] -> Matrix Concatenate/2  "P_s"
  [omega] -> Matrix Concatenate/1  "omega"
  Complex to Magnitude-Angle1/1 -> AVR_Vmeas_Filter2/1(in)  "v"
  [Q_s] -> Matrix Concatenate/4  "Q_s"
  Selector3/1 -> [Q_s_to_follow_own]
  Selector/1 -> [omega_to_follow_own]
  Selector1/1 -> Gain10/1
  Selector2/1 -> [v_to_follow_own]
  [connect] -> Memory1/1
  [connected] -> Memory/1
  Cast To Double1/1 -> Matrix Concatenate/5
  Cast To Double/1 -> Matrix Concatenate/6
  From14/1 -> Sum6/2
  Real-Imag to Complex1/1 -> Complex to Magnitude-Angle1/1
  [vdout] -> Product/1, Product2/1
  [vqout] -> Product3/1, Product1/2
  [v_d_PCC] -> Real-Imag to Complex1/1  "vod"
  [v_q_PCC] -> Real-Imag to Complex1/2  "voq"
  Sum7/1 -> Sum3/1
  connect/3(connected) -> [connected]
  [connect] -> connect/3(connect)
  connect/1(id_real) -> Real-Imag to Complex2/1, trim_output/1(id), Matrix Concatenate1/1, Product1/1, Product2/2
  Selector4/1 -> Cast To Boolean/1
  Cast To Boolean/1 -> Memory2/1
  From5/1 -> Sum8/2
  Gain8/1 -> Integrator3/1
  Gain7/1 -> Sum9/1
  Integrator3/1 -> Sum9/2
  Sum8/1 -> Gain8/1, Gain7/1
  From6/1 -> Sum8/1
  Zero1/1 -> Assignment/1
  Signal Specification/1 -> elec_out/1
  elec_in/1 -> Selector4/1, Selector3/1, Selector2/1, Selector1/1, Selector/1
  Assignment/1 -> Signal Specification/1
  Matrix Concatenate/1 -> Assignment/2
  Matrix Concatenate1/1 -> Signal Specification1/1
  Signal Specification1/1 -> For Each Subsystem/1(In1)
  Constant/1 -> Matrix Concatenate1/3
  For Each Subsystem/1(Out1) -> i/1
  connect/2(iq_real) -> Product3/2, Product/2, Real-Imag to Complex2/2, trim_output/2(iq), Matrix Concatenate1/2
  trim_output/3(Out3) -> Terminator4/1
  trim_output/1(Out1) -> Terminator2/1
  trim_output/4(Out4) -> Terminator5/1
  trim_output/2(Out2) -> Terminator3/1
  v/1 -> Selector6/1, Selector5/1
  Selector5/1 -> [vdout], trim_output/3(vd)
  Selector6/1 -> [vqout], trim_output/4(vq)
  [vqout] -> Reference frame transform3/3(in_q)
  [vdout] -> Reference frame transform3/1(in_d)
  Reference frame transform3/1(out_d) -> [v_d_PCC]
  Reference frame transform3/2(out_q) -> [v_q_PCC]
  Memory/1 -> Cast To Double/1
  Gain10/1 -> [P_s_to_follow_own]
  Memory1/1 -> Cast To Double1/1
  Memory2/1 -> [connect]
  Selector7/1 -> Sum1/2
  Selector8/1 -> Product4/2
  [omega_base] -> Selector8/1
  Product4/1 -> theta/1
  Sum1/1 -> Product4/1
  Sum3/1 -> Subsystem4/1(In1)
  Sum2/1 -> Gain/1
  Torque/1(te) -> Gain3/1
  Gain3/1 -> Rotor axis/1(te)
  Integrator1/1 -> Sum10/1
  AVR_MainRegulator/1(out) -> AVR_LeadLag/1(In1)
  AVR_Vmeas_Filter/1(out) -> Sum10/2
  AVR_Exciter/1(out) -> Gain1/1
  AVR_LeadLag/1(Out1) -> AVR_Exciter/1(in)
  From19/1 -> Real-Imag to Complex/1
  Abs/1 -> AVR_Vmeas_Filter/1(in)  "v"
  From21/1 -> Real-Imag to Complex/2
  Real-Imag to Complex/1 -> Abs/1
  Sum11/1 -> AVR_MainRegulator/1(in)
  Gain6/1 -> Sum11/1
  PIv_d1/1(vfd) -> Gain6/1
  Sum10/1 -> Scope/1, PIv_d1/1(In1)
  Gain1/1 -> Scope2/1
  AVR_Vmeas_Filter1/1(out) -> Sum2/2
  AVR_Vmeas_Filter2/1(out) -> Matrix Concatenate/3, Scope3/1
  Integrator5/1 -> Rotor axis/2(tm)
  Real-Imag to Complex2/1 -> Complex to Magnitude-Angle2/1
  Complex to Magnitude-Angle2/1 -> Scope3/2  "v"
  Electromagnetic/2(isq) -> [isq], Torque/3(isq), Reference frame transform1/3(in_q)
  Electromagnetic/1(isd) -> Reference frame transform1/1(in_d), Torque/2(isd), [isd]
  [v_d_PCC] -> Electromagnetic/1(vsd)
  [v_q_PCC] -> Electromagnetic/2(vsq)
  Integrator4/1 -> Electromagnetic/3(vfd)
  Electromagnetic/3(psi) -> Torque/1(psi)

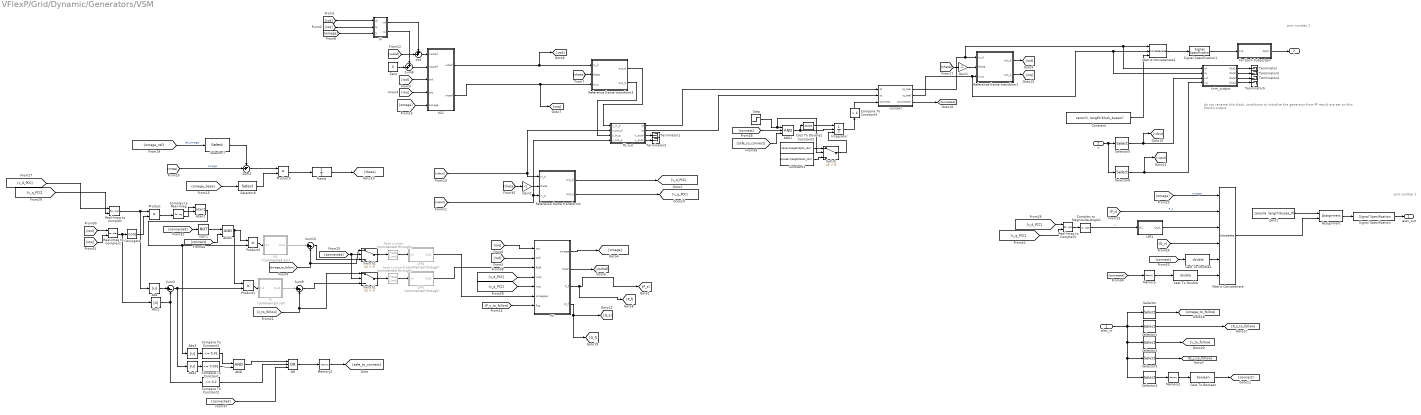
== system VFlexP/Grid/Dynamic/Generators/VSM ==
  note: port number 2
  note: do not rename this block, conditions to initialise the generator from PF result are set on this block's output
  note: port number 1
  elec_in : Inport
  v : Inport  Port=2
  AND : Logic  IconShape=distinctive  AllPortsSameDT=off  OutDataTypeStr=boolean
  AND1 : Logic  Inputs=3  IconShape=distinctive  AllPortsSameDT=off  OutDataTypeStr=boolean
  AND2 : Logic  IconShape=distinctive  AllPortsSameDT=off  OutDataTypeStr=boolean
  Abs{,1..3} (4 alike) : Abs  ZeroCross=off  SaturateOnIntegerOverflow=off
  Assignment : Assignment  NumberOfDimensions=2  DiagnosticForDimensions=Warning  IndexOptions=Assign all,Index vector (dialog)  Indices=1,block_idx  OutputSizes=1,1
  Atan2 : Trigonometry  Operator=atan2
  Cast To Boolean : DataTypeConversion  OutDataTypeStr=boolean  SaturateOnIntegerOverflow=off  RndMeth=Floor
  Cast To Double : DataTypeConversion  OutDataTypeStr=double  SaturateOnIntegerOverflow=off  RndMeth=Floor
  Cast To Double1 : DataTypeConversion  OutDataTypeStr=double  SaturateOnIntegerOverflow=off  RndMeth=Floor
  Cast To Double2 : DataTypeConversion  OutDataTypeStr=double  SaturateOnIntegerOverflow=off  RndMeth=Floor
  Compare To Constant : simulink/Logic and Bit Operations/Compare To Constant  relop=<=  const=0.001  OutDataTypeStr=boolean  ZeroCross=off
  Compare To Constant1 : simulink/Logic and Bit Operations/Compare To Constant  relop=<=  const=0.01  OutDataTypeStr=boolean  ZeroCross=off
  Compare To Constant2 : simulink/Logic and Bit Operations/Compare To Constant  relop=<=  const=0.2  OutDataTypeStr=boolean  ZeroCross=off
  Compare To Constant3 : simulink/Logic and Bit Operations/Compare To Constant  relop=>  const=4  OutDataTypeStr=boolean  ZeroCross=off
  Complex to Magnitude-Angle1 : ComplexToMagnitudeAngle  Output=Magnitude
  Complex to Real-Imag : ComplexToRealImag
  Conjugate : Math  Operator=conj  SignedPower=on  RndMeth=Zero
  Constant : Constant  Value=zeros(1, length(block_buses))  VectorParams1D=off
  Constant1 : Constant  Value=5*ones(1,length(block_idx))  VectorParams1D=off
  Constant2 : Constant  Value=zeros(1,length(block_idx))  VectorParams1D=off
  For Each Subsystem : Subsystem  TreatAsAtomicUnit=on
  Gain1 : Gain  Gain=-1
  Gain2 : Gain  Gain=-1
  Integrator : Integrator  ExternalReset=falling  InitialConditionSource=external  InitialCondition=[5]
  LPF1 : Subsystem
  LPF4 : Subsystem  Commented=through
  LPF5 : Subsystem  Commented=through
  Matrix Concatenate : Concatenate  NumInputs=6  Mode=Multidimensional array
  Matrix Concatenate1 : Concatenate  NumInputs=3  Mode=Multidimensional array
  Memory : Memory  InitialCondition=1
  Memory1 : Memory  InitialCondition=1
  Memory2 : Memory  InitialCondition=1
  NOT1 : Logic  Operator=NOT  IconShape=distinctive  AllPortsSameDT=off  OutDataTypeStr=boolean
  OR : Logic  Operator=OR  Inputs=3  IconShape=distinctive  AllPortsSameDT=off  OutDataTypeStr=boolean
  PC : Subsystem  mask(PC_VCVSC){Tf=Tf/(2*mp), mp=mp, nq=nq}
      mask prompts: Tf "Low-pass filter time constant (s)"; mp "Droop coefficient mp"; nq "Droop coefficient nq"
      mask help: Power controller of a grid-forming converter, including the droop control and low-pass filters for the power measurements.
      mask init: same as VFlexP/Grid/Dynamic/DCAC converters/DC_VCVSC/PC
  PI : Subsystem  Commented=on
  PI1 : Subsystem  Commented=on
  Product : Product
  Product1 : Product  OutDataTypeStr=double
  Product2 : Product  OutDataTypeStr=double
  Product3 : Product
  RL out : Subsystem  Variant=on  VariantControlMode=label  LabelModeActiveChoice=dynamic  mask{dynamic=Dynamic, R=R_out, L=L_out, fbase=50}
      mask prompts: dynamic "Dynamic behavior"; R "Series resistance (p.u.)"; L "Inductance (p.u.)"; fbase "Base frequency (Hz)"
      mask init: same as VFlexP/Grid/Loadflow/Generators/RL out
      mask TypeOptions dynamic: Static | Dynamic | Static omega
  Rate Limiter : RateLimiter  Commented=through  RisingSlewLimit=0.01  FallingSlewLimit=-0.01  SampleTimeMode=inherited
  Rate Limiter1 : RateLimiter  Commented=through  RisingSlewLimit=0.01  FallingSlewLimit=-0.01  SampleTimeMode=inherited
  Real-Imag to Complex : RealImagToComplex
  Real-Imag to Complex1 : RealImagToComplex
  Real-Imag to Complex3 : RealImagToComplex
  Reference frame transform1 : Subsystem
  Reference frame transform2 : Subsystem
  Reference frame transform3 : Subsystem
  Selector : Selector  NumberOfDimensions=2  InputPortWidth=3  IndexOptions=Index vector (dialog),Index vector (dialog)  Indices=1,block_idx  OutputSizes=1,1
  Selector1 : Selector  NumberOfDimensions=2  InputPortWidth=3  IndexOptions=Index vector (dialog),Index vector (dialog)  Indices=2,block_idx  OutputSizes=1,1
  Selector2 : Selector  NumberOfDimensions=2  InputPortWidth=3  IndexOptions=Index vector (dialog),Index vector (dialog)  Indices=3,block_idx  OutputSizes=1,1
  Selector3 : Selector  NumberOfDimensions=2  InputPortWidth=3  IndexOptions=Index vector (dialog),Index vector (dialog)  Indices=4,block_idx  OutputSizes=1,1
  Selector4 : Selector  NumberOfDimensions=2  InputPortWidth=3  IndexOptions=Index vector (dialog),Index vector (dialog)  Indices=5,block_idx  OutputSizes=1,1
  Selector5 : Selector  NumberOfDimensions=2  InputPortWidth=3  IndexOptions=Index vector (dialog),Index vector (dialog)  Indices=1,block_buses  OutputSizes=1,1
  Selector6 : Selector  NumberOfDimensions=2  InputPortWidth=3  IndexOptions=Index vector (dialog),Index vector (dialog)  Indices=2,block_buses  OutputSizes=1,1
  Selector7 : Selector  InputPortWidth=length(fref.ref_units)  IndexOptions=Index vector (dialog)  Indices=block_fref  OutputSizes=1
  Selector8 : Selector  InputPortWidth=length(fref.ref_units)  IndexOptions=Index vector (dialog)  Indices=block_fref  OutputSizes=1
  Signal Specification : SignalSpecification  Dimensions=[6 length(buses_lf)]
  Signal Specification1 : SignalSpecification  Dimensions=[3 length(block_buses)]
  Step : Step  Time=0.01  SampleTime=0  VectorParams1D=off  ZeroCross=off
  Sum10 : Sum  Inputs=|++
  Sum2 : Sum  Inputs=-+|
  Sum3 : Sum  Inputs=|+-
  Sum8 : Sum  Inputs=++|
  Sum9 : Sum  Inputs=|++
  Switch : Switch  Criteria=u2 > Threshold  SaturateOnIntegerOverflow=off  InputSameDT=off
  Switch1 : Switch  Criteria=u2 > Threshold  SaturateOnIntegerOverflow=off  InputSameDT=off
  Switch2 : Switch  Criteria=u2 > Threshold  SaturateOnIntegerOverflow=off  InputSameDT=off
  Terminator{,1..5} (6 alike) : Terminator
  VCC : Subsystem  Variant=on  VariantControlMode=label  LabelModeActiveChoice=dynamic
  VI : Subsystem  mask{L=VI_L, R=VI_R, Tf=WOF_Tf}
      mask prompts: L "Inductance (pu)"; R "Resistance (pu)"; Tf "WOF time constant (s)"
      mask init: same as VFlexP/Grid/Dynamic/DCAC converters/DC_VCVSC/VI
  Zero : Constant  Value=0  OutDataTypeStr=Inherit: Inherit via back propagation
  Zero1 : Constant  Value=zeros(6, length(buses_lf))  VectorParams1D=off  OutDataTypeStr=Inherit: Inherit via back propagation
  connect : Subsystem
  frame : Integrator  InitialCondition=Grid_op_VSM.op.States(17).x'  IgnoreLimit=on
  trim_output : Subsystem
  vod : Sum  Inputs=++|
  elec_out : Outport
  i : Outport  Port=2
  wires:
  VCC/2(viqref) -> Reference frame transform3/3(in_q), [voq]
  VCC/1(vidref) -> Reference frame transform3/1(in_d), [vod]
  Memory1/1 -> Cast To Boolean/1
  Switch/1 -> Integrator/3
  Cast To Double2/1 -> Integrator/1
  AND1/1 -> Integrator/2, Cast To Double2/1
  [safe_to_connect] -> AND1/3
  Constant1/1 -> Switch/3
  Step/1 -> AND1/1, Switch/2
  Constant2/1 -> Switch/1
  Integrator/1 -> Compare To Constant3/1
  [connect] -> AND1/2
  AND2/1 -> Product2/1, Product1/1
  [connect] -> AND2/2
  [connected] -> NOT1/1
  NOT1/1 -> AND2/1
  [omega_to_follow] -> Sum10/2, Switch2/1
  Selector1/1 -> [P_s_to_follow]
  Memory/1 -> Cast To Double/1
  Selector5/1 -> trim_output/3(vd), [vdout]
  Selector6/1 -> trim_output/4(vq), [vqout]
  v/1 -> Selector5/1, Selector6/1
  trim_output/4(Out4) -> Terminator5/1
  trim_output/3(Out3) -> Terminator4/1
  trim_output/2(Out2) -> Terminator3/1
  trim_output/1(Out1) -> Terminator/1
  Zero1/1 -> Assignment/1
  [v_d_PCC] -> Real-Imag to Complex3/1
  [v_q_PCC] -> Real-Imag to Complex3/2
  Real-Imag to Complex3/1 -> Complex to Magnitude-Angle1/1
  [v_q_PCC] -> PC/5(voq)
  [v_d_PCC] -> PC/4(vodi)
  Signal Specification1/1 -> For Each Subsystem/1(In1)
  For Each Subsystem/1(Out1) -> i/1
  Constant/1 -> Matrix Concatenate1/3
  Matrix Concatenate1/1 -> Signal Specification1/1
  [vdout] -> Reference frame transform2/1(in_d), RL out/2(v_out_d)
  Reference frame transform2/2(out_q) -> [v_q_PCC]
  Reference frame transform2/1(out_d) -> [v_d_PCC]
  [vqout] -> RL out/4(v_out_q), Reference frame transform2/3(in_q)
  Memory2/1 -> [safe_to_connect]
  [connected] -> OR/3
  Compare To Constant2/1 -> OR/2
  OR/1 -> Memory2/1
  AND/1 -> OR/1
  Compare To Constant1/1 -> AND/1
  Abs3/1 -> Compare To Constant1/1
  Compare To Constant/1 -> AND/2
  Abs2/1 -> Compare To Constant/1
  Signal Specification/1 -> elec_out/1
  Abs1/1 -> Sum3/2, Compare To Constant2/1
  Cast To Boolean/1 -> [connect]
  Switch2/1 -> Rate Limiter/1
  PI1/1(Out1) -> Sum10/1
  Atan2/1 -> Product2/2, Abs3/1
  Product2/1 -> PI1/1(In1)
  Product1/1 -> PI/1(In1)
  PI/1(Out1) -> Sum9/1
  Sum3/1 -> Product1/2, Abs2/1
  Abs/1 -> Sum3/1
  Complex to Real-Imag/1 -> Atan2/2
  Complex to Real-Imag/2 -> Atan2/1
  Product/1 -> Complex to Real-Imag/1
  Conjugate/1 -> Product/2
  Real-Imag to Complex/1 -> Product/1, Abs/1
  Real-Imag to Complex1/1 -> Conjugate/1, Abs1/1
  [voq] -> Real-Imag to Complex1/2
  [vod] -> Real-Imag to Complex1/1
  [v_q_PCC] -> Real-Imag to Complex/2
  [v_d_PCC] -> Real-Imag to Complex/1
  Cast To Double1/1 -> Matrix Concatenate/5
  Cast To Double/1 -> Matrix Concatenate/6
  Selector4/1 -> Memory1/1
  [connected] -> Memory/1
  [connect] -> Cast To Double1/1
  Assignment/1 -> Signal Specification/1
  elec_in/1 -> Selector/1, Selector1/1, Selector2/1, Selector3/1, Selector4/1
  Matrix Concatenate/1 -> Assignment/2
  [omega] -> Matrix Concatenate/1  "omega"
  Complex to Magnitude-Angle1/1 -> LPF1/1(In1)  "v"
  [P_s] -> Matrix Concatenate/2  "P_s"
  [Q_s] -> Matrix Concatenate/4
  Selector2/1 -> [v_to_follow]
  Selector/1 -> [omega_to_follow]
  Selector3/1 -> [Q_s_to_follow]
  RL out/4(v_outq) -> Terminator2/1
  RL out/3(v_outd) -> Terminator1/1
  connect/2(iq_real) -> Reference frame transform1/3(in_q), Matrix Concatenate1/2, trim_output/2(iq)
  connect/1(id_real) -> Reference frame transform1/1(in_d), Matrix Concatenate1/1, trim_output/1(id)
  VI/2(vq) -> Sum8/1
  VI/1(vd) -> vod/1
  Reference frame transform1/1(out_d) -> [iod]
  RL out/2(iq) -> connect/2(iq)
  Reference frame transform3/2(out_q) -> RL out/3(v_in_q)
  Reference frame transform3/1(out_d) -> RL out/1(v_in_d)
  Reference frame transform1/2(out_q) -> [ioq]
  [ioq] -> PC/1(ioq)
  [iod] -> PC/2(iodi)
  PC/2(Out2) -> [vodref]
  PC/1(omega) -> [omega]
  [theta] -> Reference frame transform3/2(theta)
  [omega] -> VCC/5(omega)
  [vodref] -> vod/2
  Zero/1 -> Sum8/2
  [iod] -> VCC/3(iod)
  [ioq] -> VCC/4(ioq)
  Gain1/1 -> Reference frame transform1/2(theta)
  [theta] -> Gain1/1
  RL out/1(id) -> connect/1(id)
  Sum2/1 -> Product3/1
  [omega_ref] -> Selector7/1  "ref_omega"
  [omega] -> Sum2/2  "omega"
  connect/3(connected) -> [connected]
  PC/3(P_f) -> [P_f], [P_s]
  PC/4(Q_f) -> [Q_f], [Q_s]
  [P_s_to_follow] -> PC/7(Psp)
  frame/1 -> [theta]
  Product3/1 -> frame/1
  Rate Limiter1/1 -> LPF5/1(In1)
  [theta] -> Gain2/1
  Gain2/1 -> Reference frame transform2/2(theta)
  [iod] -> VI/1(id)
  [ioq] -> VI/2(iq)
  [omega] -> VI/3(omega)
  vod/1 -> VCC/1(vodref)
  Sum8/1 -> VCC/2(voqref)
  Rate Limiter/1 -> LPF4/1(In1)
  Sum10/1 -> Switch2/3
  Sum9/1 -> Switch1/3
  [connected] -> Switch1/2, Switch2/2
  Switch1/1 -> Rate Limiter1/1
  [v_to_follow] -> Sum9/2, Switch1/1
  LPF4/1(Out1) -> PC/6(omegasp)
  LPF5/1(Out1) -> PC/3(Eref)
  Selector7/1 -> Sum2/1
  [omega_base] -> Selector8/1
  Selector8/1 -> Product3/2
  LPF1/1(Out1) -> Matrix Concatenate/3
  Compare To Constant3/1 -> connect/3(connect)

== system VFlexP/Grid/Dynamic/Generators_DC/DCBUCK ==
  v : Inport
  ref : Inport  Port=2
  Constant2 : Constant  Value=block_Pg./(DC.v(block_buses)*Sb)  VectorParams1D=off
  Gain : Gain  Gain=0.6
  Gain1 : Gain  Gain=565.4867
  Gain4 : Gain  Gain=1/1.5915e-04
  Gain5 : Gain  Gain=0.01
  Integrator : Integrator  InitialCondition=Grid_DCop_DCBUCK.op.States(1).x'
  Integrator1 : Integrator  InitialCondition=Grid_DCop_DCBUCK.op.States(2).x'
  Selector : Selector  InputPortWidth=DC.Nbuses  IndexOptions=Index vector (dialog)  Indices=block_buses  OutputSizes=1
  Selector1 : Selector  Commented=on  InputPortWidth=3  IndexOptions=Index vector (dialog)  Indices=[1 3]  OutputSizes=1
  State-Space : StateSpace  A=[]  B=[]  C=[]  D=block_toM  InitialCondition=0  ParameterTunability=Optimized
  Sum : Sum  Inputs=|++
  Sum2 : Sum  Inputs=|+-
  Sum3 : Sum  Inputs=++-
  Transpose : Math  Operator=transpose
  Transpose1 : Math  Operator=transpose
  i : Outport
  wires:
  Gain5/1 -> Sum3/3
  Selector/1 -> Sum3/1
  v/1 -> Selector/1
  ref/1 -> Selector1/1
  Constant2/1 -> Sum2/1
  Sum3/1 -> Gain4/1
  Transpose1/1 -> i/1
  Sum2/1 -> Gain/1, Gain1/1
  Gain4/1 -> Integrator/1
  Integrator1/1 -> Sum/1
  Gain/1 -> Sum/2
  Sum/1 -> Sum3/2
  Gain1/1 -> Integrator1/1
  Transpose/1 -> State-Space/1
  Integrator/1 -> Transpose/1, Gain5/1, Sum2/2
  State-Space/1 -> Transpose1/1
